simulink model "lab5 (2)"  (R2021a)
settings: Solver=VariableStepAuto  StartTime=0.0  StopTime=10  MaxStep=0.01  RelTol=1e-3
libraries: simulink_extras x2
settings Model: Creator=kaa040803  LastModifiedBy=error
settings SolverCC: AlgebraicLoopSolver=TrustRegion
settings DebuggingCC: SFMachineParentedDataDiag=warning

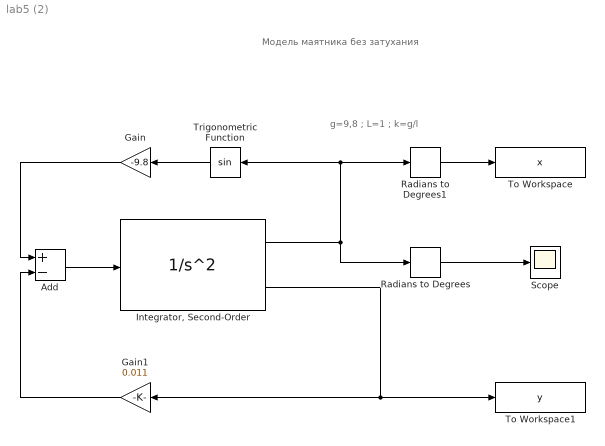
== system lab5 (2) ==
  note: Модель маятника без затухания
  note: g=9,8 ; L=1 ; k=g/l
  Add : Sum  Inputs=+-
  Gain : Gain  Gain=-9.8
  Gain1 : Gain  Gain=0.011
  "Integrator, Second-Order" : SecondOrderIntegrator  ICX=2*pi/3+0.011
  Radians to Degrees : simulink_extras/Transformations/Radians to Degrees
  Radians to Degrees1 : simulink_extras/Transformations/Radians to Degrees
  Scope : Scope
  To Workspace : ToWorkspace  VariableName=x  SampleTime=-1
  To Workspace1 : ToWorkspace  VariableName=y  SampleTime=-1
  Trigonometric Function : Trigonometry
  wires:
  Trigonometric Function/1 -> Gain/1
  Add/1 -> "Integrator, Second-Order"/1
  Gain/1 -> Add/1
  Gain1/1 -> Add/2
  "Integrator, Second-Order"/2 -> To Workspace1/1, Gain1/1
  Radians to Degrees/1 -> Scope/1
  Radians to Degrees1/1 -> To Workspace/1
  "Integrator, Second-Order"/1 -> Radians to Degrees1/1, Trigonometric Function/1, Radians to Degrees/1
